simulink library "CAN_PT_lib"  (Simulink 7.5)
settings: Solver=ode45  StartTime=0.0  StopTime=10.0  RelTol=1e-3
undefined symbols (not defined in the file): p_bool_False_M, pOUTP_pct_BatSOCIC_CUR, pOUTP_pct_BatSOCLim_C, pOUTP_pct_BatSOCRaw_TAB, pOUTP_st_ACPTCfg_C, pOUTP_st_ChrgrPlugStOne_C, pOUTP_st_ChrgrPlugStTwo_C, pOUTP_st_ChrgrPlugStZero_C, pOUTP_st_DCDCErrSt_C, pOUTP_st_EVRdyNoSt_C, pOUTP_st_EVRdyRdySt_C, pOUTP_st_HCUStNoErr_C, pOUTP_w_OutPwrCvrt_C, pOUTP_w_OutPwrGenrMax_C, pOUTP_w_OutPwrMax_C, VMMCoorrStsTyp
libraries: BaseOperationLib_Browser x40, PES_CZ_FAW x1, simulink x1
settings Model: Creator=wuaibin  LastModifiedBy=wuaibin

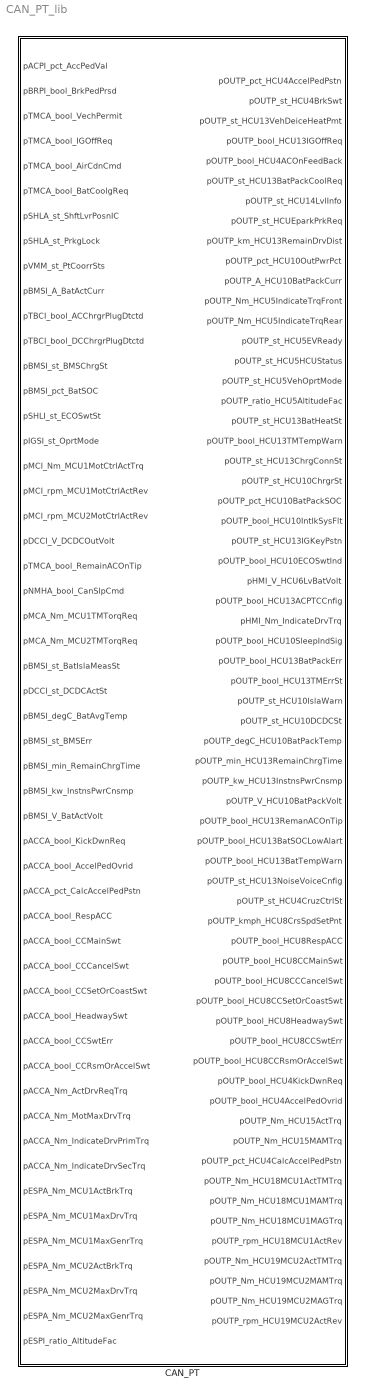
== system CAN_PT_lib ==
  CAN_PT : Subsystem  TreatAsAtomicUnit=on

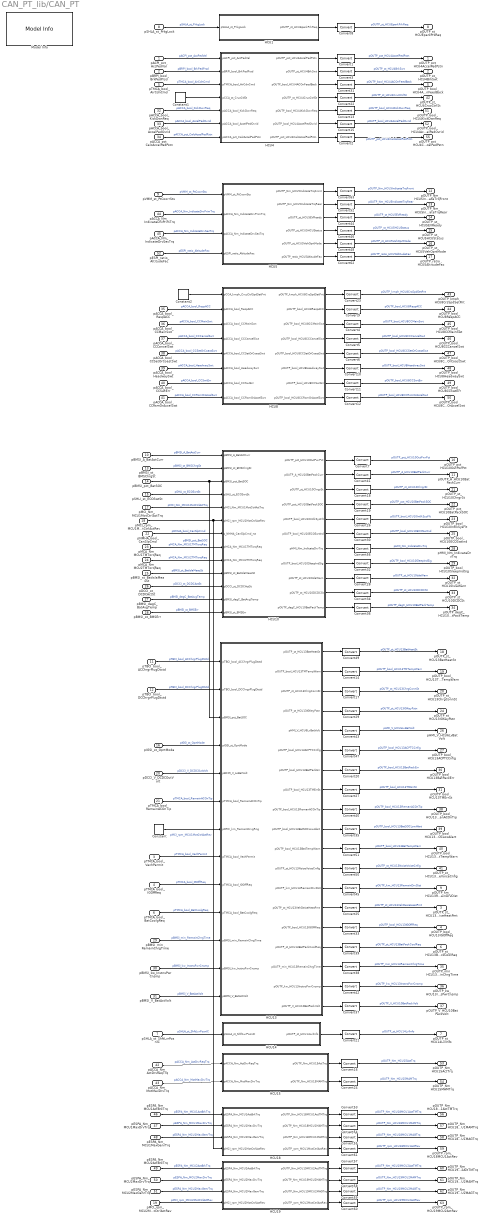
== system CAN_PT_lib/CAN_PT ==
  pACPI_pct_AccPedVal : Inport  OutDataType=fixdt(1, 16)  OutScaling=2^0
  pBRPI_bool_BrkPedPrsd : Inport  Port=2  OutDataType=fixdt(1, 16)  OutScaling=2^0
  pTMCA_bool_VechPermit : Inport  Port=3  OutDataType=fixdt(1, 16)  OutScaling=2^0
  pTMCA_bool_IGOffReq : Inport  Port=4  OutDataType=fixdt(1, 16)  OutScaling=2^0
  pTMCA_bool_AirCdnCmd : Inport  Port=5  OutDataType=fixdt(1, 16)  OutScaling=2^0
  pTMCA_bool_BatCoolgReq : Inport  Port=6  OutDataType=fixdt(1, 16)  OutScaling=2^0
  pSHLA_st_ShftLvrPosnIC : Inport  Port=7  OutDataType=fixdt(1, 16)  OutScaling=2^0
  pSHLA_st_PrkgLock : Inport  Port=8  OutDataType=fixdt(1, 16)  OutScaling=2^0
  pVMM_st_PtCoorrSts : Inport  Port=9
  pBMSI_A_BatActCurr : Inport  Port=10
  pTBCI_bool_ACChrgrPlugDtctd : Inport  Port=11
  pTBCI_bool_DCChrgrPlugDtctd : Inport  Port=12
  pBMSI_st_BMSChrgSt : Inport  Port=13
  pBMSI_pct_BatSOC : Inport  Port=14
  pSHLI_st_ECOSwtSt : Inport  Port=15
  pIGSI_st_OprtMode : Inport  Port=16
  pMCI_Nm_MCU1MotCtrlActTrq : Inport  Port=17
  pMCI_rpm_MCU1MotCtrlActRev : Inport  Port=18
  pMCI_rpm_MCU2MotCtrlActRev : Inport  Port=19
  pDCCI_V_DCDCOutVolt : Inport  Port=20
  pTMCA_bool_RemainACOnTip : Inport  Port=21
  pNMHA_bool_CanSlpCmd : Inport  Port=22  OutDataType=fixdt(1, 16)  OutScaling=2^0
  pMCA_Nm_MCU1TMTorqReq : Inport  Port=23
  pMCA_Nm_MCU2TMTorqReq : Inport  Port=24
  pBMSI_st_BatIslaMeasSt : Inport  Port=25
  pDCCI_st_DCDCActSt : Inport  Port=26
  pBMSI_degC_BatAvgTemp : Inport  Port=27
  pBMSI_st_BMSErr : Inport  Port=28
  pBMSI_min_RemainChrgTime : Inport  Port=29
  pBMSI_kw_InstnsPwrCnsmp : Inport  Port=30
  pBMSI_V_BatActVolt : Inport  Port=31
  pACCA_bool_KickDwnReq : Inport  Port=32  OutDataType=fixdt(1, 16)  OutScaling=2^0
  pACCA_bool_AccelPedOvrid : Inport  Port=33  OutDataType=fixdt(1, 16)  OutScaling=2^0
  pACCA_pct_CalcAccelPedPstn : Inport  Port=34  OutDataType=fixdt(1, 16)  OutScaling=2^0
  pACCA_bool_RespACC : Inport  Port=35
  pACCA_bool_CCMainSwt : Inport  Port=36
  pACCA_bool_CCCancelSwt : Inport  Port=37
  pACCA_bool_CCSetOrCoastSwt : Inport  Port=38
  pACCA_bool_HeadwaySwt : Inport  Port=39
  pACCA_bool_CCSwtErr : Inport  Port=40
  pACCA_bool_CCRsmOrAccelSwt : Inport  Port=41
  pACCA_Nm_ActDrvReqTrq : Inport  Port=42  OutDataType=fixdt(1, 16)  OutScaling=2^0
  pACCA_Nm_MotMaxDrvTrq : Inport  Port=43  OutDataType=fixdt(1, 16)  OutScaling=2^0
  pACCA_Nm_IndicateDrvPrimTrq : Inport  Port=44  OutDataType=fixdt(1, 16)  OutScaling=2^0
  pACCA_Nm_IndicateDrvSecTrq : Inport  Port=45  OutDataType=fixdt(1, 16)  OutScaling=2^0
  pESPA_Nm_MCU1ActBrkTrq : Inport  Port=46  OutDataType=fixdt(1, 16)  OutScaling=2^0
  pESPA_Nm_MCU1MaxDrvTrq : Inport  Port=47  OutDataType=fixdt(1, 16)  OutScaling=2^0
  pESPA_Nm_MCU1MaxGenrTrq : Inport  Port=48  OutDataType=fixdt(1, 16)  OutScaling=2^0
  pESPA_Nm_MCU2ActBrkTrq : Inport  Port=49  OutDataType=fixdt(1, 16)  OutScaling=2^0
  pESPA_Nm_MCU2MaxDrvTrq : Inport  Port=50  OutDataType=fixdt(1, 16)  OutScaling=2^0
  pESPA_Nm_MCU2MaxGenrTrq : Inport  Port=51  OutDataType=fixdt(1, 16)  OutScaling=2^0
  pESPI_ratio_AltitudeFac : Inport  Port=52  OutDataType=fixdt(1, 16)  OutScaling=2^0
  Constant : BaseOperationLib_Browser/Sources&Sinks/Constant  Value=0  OutMin=[]  OutMax=[]  OutDataType=fixdt(1, 16)  ConRadixGroup=Use specified scaling  OutScaling=2^0  OutDataTypeStr=Inherit: Inherit from 'Constant value'
  Constant1 : BaseOperationLib_Browser/Sources&Sinks/Constant  Value=0  OutMin=[]  OutMax=[]  OutDataType=fixdt(1, 16)  ConRadixGroup=Use specified scaling  OutScaling=2^0  OutDataTypeStr=Inherit: Inherit from 'Constant value'
  Constant2 : BaseOperationLib_Browser/Sources&Sinks/Constant  Value=0  OutMin=[]  OutMax=[]  OutDataType=fixdt(1, 16)  ConRadixGroup=Use specified scaling  OutScaling=2^0  OutDataTypeStr=Inherit: Inherit from 'Constant value'
  Convert{1..63} (63 alike) : DataTypeConversion  OutDataType=fixdt(1, 16)  OutScaling=2^0
  HCU1 : Subsystem
  HCU10 : Subsystem
  HCU13 : Subsystem
  HCU14 : Subsystem
  HCU15 : Subsystem
  HCU18 : Subsystem
  HCU19 : Subsystem
  HCU4 : Subsystem
  HCU5 : Subsystem
  HCU8 : Subsystem
  Model Info : simulink/Model-Wide Utilities/Model Info  SystemSampleTime=-1  InitialBlockCM=None  BlockCM=None  Frame=on  DisplayStringWithTags=Model Info\nCreated: %<Created>\nCreator: wuaibin  HorizontalTextAlignment=Center  LeftAlignmentValue=0.5  SourceBlockDiagram=HQEV_HCU  TagMaxNumber=20
  pOUTP_pct_HCU4AccelPedPstn : Outport  OutDataType=fixdt(1, 16)  OutScaling=2^0
  pOUTP_st_HCU4BrkSwt : Outport  Port=2  OutDataType=fixdt(1, 16)  OutScaling=2^0
  pOUTP_st_HCU13VehDeiceHeatPmt : Outport  Port=3  OutDataType=fixdt(1, 16)  OutScaling=2^0
  pOUTP_bool_HCU13IGOffReq : Outport  Port=4  OutDataType=fixdt(1, 16)  OutScaling=2^0
  pOUTP_bool_HCU4ACOnFeedBack : Outport  Port=5  OutDataType=fixdt(1, 16)  OutScaling=2^0
  pOUTP_st_HCU13BatPackCoolReq : Outport  Port=6  OutDataType=fixdt(1, 16)  OutScaling=2^0
  pOUTP_st_HCU14LvlInfo : Outport  Port=7  OutDataType=fixdt(1, 16)  OutScaling=2^0
  pOUTP_st_HCUEparkPrkReq : Outport  Port=8  OutDataType=fixdt(1, 16)  OutScaling=2^0
  pOUTP_km_HCU13RemainDrvDist : Outport  Port=9  OutDataType=fixdt(1, 16)  OutScaling=2^0
  pOUTP_pct_HCU10OutPwrPct : Outport  Port=10
  pOUTP_A_HCU10BatPackCurr : Outport  Port=11
  pOUTP_Nm_HCU5IndicateTrqFront : Outport  Port=12
  pOUTP_Nm_HCU5IndicateTrqRear : Outport  Port=13
  pOUTP_st_HCU5EVReady : Outport  Port=14
  pOUTP_st_HCU5HCUStatus : Outport  Port=15
  pOUTP_st_HCU5VehOprtMode : Outport  Port=16
  pOUTP_ratio_HCU5AltitudeFac : Outport  Port=17
  pOUTP_st_HCU13BatHeatSt : Outport  Port=18
  pOUTP_bool_HCU13TMTempWarn : Outport  Port=19
  pOUTP_st_HCU13ChrgConnSt : Outport  Port=20
  pOUTP_st_HCU10ChrgrSt : Outport  Port=21
  pOUTP_pct_HCU10BatPackSOC : Outport  Port=22
  pOUTP_bool_HCU10IntlkSysFlt : Outport  Port=23
  pOUTP_st_HCU13IGKeyPstn : Outport  Port=24
  pOUTP_bool_HCU10ECOSwtInd : Outport  Port=25
  pHMI_V_HCU6LvBatVolt : Outport  Port=26
  pOUTP_bool_HCU13ACPTCCnfig : Outport  Port=27
  pHMI_Nm_IndicateDrvTrq : Outport  Port=28
  pOUTP_bool_HCU10SleepIndSig : Outport  Port=29
  pOUTP_bool_HCU13BatPackErr : Outport  Port=30
  pOUTP_bool_HCU13TMErrSt : Outport  Port=31
  pOUTP_st_HCU10IslaWarn : Outport  Port=32
  pOUTP_st_HCU10DCDCSt : Outport  Port=33
  pOUTP_degC_HCU10BatPackTemp : Outport  Port=34
  pOUTP_min_HCU13RemainChrgTime : Outport  Port=35
  pOUTP_kw_HCU13InstnsPwrCnsmp : Outport  Port=36
  pOUTP_V_HCU10BatPackVolt : Outport  Port=37
  pOUTP_bool_HCU13RemanACOnTip : Outport  Port=38  OutDataType=fixdt(1, 16)  OutScaling=2^0
  pOUTP_bool_HCU13BatSOCLowAlart : Outport  Port=39
  pOUTP_bool_HCU13BatTempWarn : Outport  Port=40  OutDataType=fixdt(1, 16)  OutScaling=2^0
  pOUTP_st_HCU13NoiseVoiceCnfig : Outport  Port=41  OutDataType=fixdt(1, 16)  OutScaling=2^0
  pOUTP_st_HCU4CruzCtrlSt : Outport  Port=42  OutDataType=fixdt(1, 16)  OutScaling=2^0
  pOUTP_kmph_HCU8CrsSpdSetPnt : Outport  Port=43  OutDataType=fixdt(1, 16)  OutScaling=2^0
  pOUTP_bool_HCU8RespACC : Outport  Port=44  OutDataType=fixdt(1, 16)  OutScaling=2^0
  pOUTP_bool_HCU8CCMainSwt : Outport  Port=45  OutDataType=fixdt(1, 16)  OutScaling=2^0
  pOUTP_bool_HCU8CCCancelSwt : Outport  Port=46  OutDataType=fixdt(1, 16)  OutScaling=2^0
  pOUTP_bool_HCU8CCSetOrCoastSwt : Outport  Port=47  OutDataType=fixdt(1, 16)  OutScaling=2^0
  pOUTP_bool_HCU8HeadwaySwt : Outport  Port=48  OutDataType=fixdt(1, 16)  OutScaling=2^0
  pOUTP_bool_HCU8CCSwtErr : Outport  Port=49  OutDataType=fixdt(1, 16)  OutScaling=2^0
  pOUTP_bool_HCU8CCRsmOrAccelSwt : Outport  Port=50  OutDataType=fixdt(1, 16)  OutScaling=2^0
  pOUTP_bool_HCU4KickDwnReq : Outport  Port=51
  pOUTP_bool_HCU4AccelPedOvrid : Outport  Port=52
  pOUTP_Nm_HCU15ActTrq : Outport  Port=53
  pOUTP_Nm_HCU15MAMTrq : Outport  Port=54
  pOUTP_pct_HCU4CalcAccelPedPstn : Outport  Port=55  OutDataType=fixdt(1, 16)  OutScaling=2^0
  pOUTP_Nm_HCU18MCU1ActTMTrq : Outport  Port=56
  pOUTP_Nm_HCU18MCU1MAMTrq : Outport  Port=57
  pOUTP_Nm_HCU18MCU1MAGTrq : Outport  Port=58
  pOUTP_rpm_HCU18MCU1ActRev : Outport  Port=59
  pOUTP_Nm_HCU19MCU2ActTMTrq : Outport  Port=60
  pOUTP_Nm_HCU19MCU2MAMTrq : Outport  Port=61
  pOUTP_Nm_HCU19MCU2MAGTrq : Outport  Port=62
  pOUTP_rpm_HCU19MCU2ActRev : Outport  Port=63
  wires:
  HCU15/2(pOUTP_Nm_HCU15MAMTrq) -> Convert24/1
  HCU15/1(pOUTP_Nm_HCU15ActTrq) -> Convert16/1
  HCU4/7(pOUTP_pct_HCU4CalcAccelPedPstn) -> Convert2/1
  HCU4/6(pOUTP_bool_HCU4AccelPedOvrid) -> Convert15/1
  HCU4/5(pOUTP_bool_HCU4KickDwnReq) -> Convert13/1
  HCU4/4(pOUTP_st_HCU4CruzCtrlSt) -> Convert22/1
  HCU13/19(pOUTP_V_HCU10BatPackVolt) -> Convert37/1
  HCU13/18(pOUTP_kw_HCU13InstnsPwrCnsmp) -> Convert42/1
  HCU13/17(pOUTP_min_HCU13RemainChrgTime) -> Convert38/1
  HCU10/11(pOUTP_degC_HCU10BatPackTemp) -> Convert36/1
  HCU10/10(pOUTP_st_HCU10DCDCSt) -> Convert34/1
  HCU10/9(pOUTP_st_HCU10IslaWarn) -> Convert28/1
  Constant/1 -> HCU13/7(pDRC_km_RemainDrvgRng)
  Convert49/1 -> pOUTP_st_HCU13BatHeatSt/1  "pOUTP_st_HCU13BatHeatSt"
  Convert14/1 -> pOUTP_bool_HCU13TMTempWarn/1  "pOUTP_bool_HCU13TMTempWarn"
  Convert17/1 -> pOUTP_st_HCU13ChrgConnSt/1  "pOUTP_st_HCU13ChrgConnSt"
  HCU13/5(pHMI_V_HCU6LvBatVolt) -> Convert43/1
  HCU5/5(pOUTP_st_HCU5VehOprtMode) -> Convert48/1
  HCU5/4(pOUTP_st_HCU5HCUStatus) -> Convert46/1
  HCU5/3(pOUTP_st_HCU5EVReady) -> Convert44/1
  HCU13/6(pOUTP_bool_HCU13ACPTCCnfig) -> Convert47/1
  HCU13/4(pOUTP_st_HCU13IGKeyPstn) -> Convert29/1
  HCU13/3(pOUTP_st_HCU13ChrgConnSt) -> Convert17/1
  HCU13/2(pOUTP_bool_HCU13TMTempWarn) -> Convert14/1
  HCU13/1(pOUTP_st_HCU13BatHeatSt) -> Convert49/1
  HCU13/13(pOUTP_km_HCU13RemainDrvDist) -> Convert45/1
  HCU13/12(pOUTP_st_HCU13NoiseVoiceCnfig) -> Convert50/1
  HCU13/11(pOUTP_bool_HCU13BatTempWarn) -> Convert51/1
  HCU13/10(pOUTP_bool_HCU13BatSOCLowAlart) -> Convert35/1
  HCU13/9(pOUTP_bool_HCU13RemanACOnTip) -> Convert40/1
  HCU13/8(pOUTP_bool_HCU13TMErrSt) -> Convert27/1
  HCU13/7(pOUTP_bool_HCU13BatPackErr) -> Convert20/1
  pSHLA_st_PrkgLock/1 -> HCU1/1(pSHLA_st_PrkgLock)  "pSHLA_st_PrkgLock"
  HCU1/1(pOUTP_st_HCUEparkPrkReq) -> Convert8/1
  pSHLA_st_ShftLvrPosnIC/1 -> HCU14/1(pSHLA_st_ShftLvrPosnIC)  "pSHLA_st_ShftLvrPosnIC"
  HCU14/1(pOUTP_st_HCU14LvlInfo) -> Convert21/1
  pTMCA_bool_AirCdnCmd/1 -> HCU4/3(pTMCA_bool_AirCdnCmd)  "pTMCA_bool_AirCdnCmd"
  HCU4/3(pOUTP_bool_HCU4ACOnFeedBack) -> Convert31/1
  pBRPI_bool_BrkPedPrsd/1 -> HCU4/2(pBRPI_bool_BrkPedPrsd)  "pBRPI_bool_BrkPedPrsd"
  pACPI_pct_AccPedVal/1 -> HCU4/1(pACPI_pct_AccPedVal)  "pACPI_pct_AccPedVal"
  HCU4/2(pOUTP_st_HCU4BrkSwt) -> Convert3/1
  HCU4/1(pOUTP_pct_HCU4AccelPedPstn) -> Convert1/1
  pMCA_Nm_MCU1TMTorqReq/1 -> HCU10/8(pMCA_Nm_MCU1TMTorqReq)  "pMCA_Nm_MCU1TMTorqReq"
  pMCA_Nm_MCU2TMTorqReq/1 -> HCU10/9(pMCA_Nm_MCU2TMTorqReq)  "pMCA_Nm_MCU2TMTorqReq"
  Constant2/1 -> HCU8/1(pCCA_kmph_CruzCtrlSpdSetPnt)
  Convert2/1 -> pOUTP_pct_HCU4CalcAccelPedPstn/1  "pOUTP_pct_HCU4CalcAccelPedPstn"
  Convert24/1 -> pOUTP_Nm_HCU15MAMTrq/1  "pOUTP_Nm_HCU15MAMTrq"
  Convert16/1 -> pOUTP_Nm_HCU15ActTrq/1  "pOUTP_Nm_HCU15ActTrq"
  Convert15/1 -> pOUTP_bool_HCU4AccelPedOvrid/1  "pOUTP_bool_HCU4AccelPedOvrid"
  Convert13/1 -> pOUTP_bool_HCU4KickDwnReq/1  "pOUTP_bool_HCU4KickDwnReq"
  HCU8/8(pOUTP_bool_HCU8CCRsmOrAccelSwt) -> Convert12/1
  HCU8/7(pOUTP_bool_HCU8CCSwtErr) -> Convert11/1
  HCU8/6(pOUTP_bool_HCU8HeadwaySwt) -> Convert10/1
  HCU8/5(pOUTP_bool_HCU8CCSetOrCoastSwt) -> Convert6/1
  HCU8/4(pOUTP_bool_HCU8CCCancelSwt) -> Convert5/1
  HCU8/3(pOUTP_bool_HCU8CCMainSwt) -> Convert4/1
  HCU8/2(pOUTP_bool_HCU8RespACC) -> Convert9/1
  HCU8/1(pOUTP_kmph_HCU8CrsSpdSetPnt) -> Convert23/1
  Convert6/1 -> pOUTP_bool_HCU8CCSetOrCoastSwt/1  "pOUTP_bool_HCU8CCSetOrCoastSwt"
  Convert5/1 -> pOUTP_bool_HCU8CCCancelSwt/1  "pOUTP_bool_HCU8CCCancelSwt"
  Convert4/1 -> pOUTP_bool_HCU8CCMainSwt/1  "pOUTP_bool_HCU8CCMainSwt"
  Convert12/1 -> pOUTP_bool_HCU8CCRsmOrAccelSwt/1  "pOUTP_bool_HCU8CCRsmOrAccelSwt"
  Convert11/1 -> pOUTP_bool_HCU8CCSwtErr/1  "pOUTP_bool_HCU8CCSwtErr"
  Convert10/1 -> pOUTP_bool_HCU8HeadwaySwt/1  "pOUTP_bool_HCU8HeadwaySwt"
  Convert9/1 -> pOUTP_bool_HCU8RespACC/1  "pOUTP_bool_HCU8RespACC"
  Convert23/1 -> pOUTP_kmph_HCU8CrsSpdSetPnt/1  "pOUTP_kmph_HCU8CrsSpdSetPnt"
  Convert22/1 -> pOUTP_st_HCU4CruzCtrlSt/1  "pOUTP_st_HCU4CruzCtrlSt"
  Convert51/1 -> pOUTP_bool_HCU13BatTempWarn/1  "pOUTP_bool_HCU13BatTempWarn"
  Convert50/1 -> pOUTP_st_HCU13NoiseVoiceCnfig/1  "pOUTP_st_HCU13NoiseVoiceCnfig"
  Convert35/1 -> pOUTP_bool_HCU13BatSOCLowAlart/1  "pOUTP_bool_HCU13BatSOCLowAlart"
  HCU10/7(pHMI_Nm_IndicateDrvTrq) -> Convert56/1
  Convert56/1 -> pHMI_Nm_IndicateDrvTrq/1  "pHMI_Nm_IndicateDrvTrq"
  HCU10/1(pOUTP_pct_HCU10OutPwrPct) -> Convert7/1
  Convert7/1 -> pOUTP_pct_HCU10OutPwrPct/1  "pOUTP_pct_HCU10OutPwrPct"
  Convert41/1 -> pOUTP_A_HCU10BatPackCurr/1  "pOUTP_A_HCU10BatPackCurr"
  HCU10/2(pOUTP_A_HCU10BatPackCurr) -> Convert41/1
  Convert44/1 -> pOUTP_st_HCU5EVReady/1  "pOUTP_st_HCU5EVReady"
  Convert46/1 -> pOUTP_st_HCU5HCUStatus/1  "pOUTP_st_HCU5HCUStatus"
  Convert48/1 -> pOUTP_st_HCU5VehOprtMode/1  "pOUTP_st_HCU5VehOprtMode"
  HCU10/3(pOUTP_st_HCU10ChrgrSt) -> Convert18/1
  Convert18/1 -> pOUTP_st_HCU10ChrgrSt/1  "pOUTP_st_HCU10ChrgrSt"
  HCU10/4(pOUTP_pct_HCU10BatPackSOC) -> Convert19/1
  Convert19/1 -> pOUTP_pct_HCU10BatPackSOC/1  "pOUTP_pct_HCU10BatPackSOC"
  Convert26/1 -> pOUTP_bool_HCU10IntlkSysFlt/1  "pOUTP_bool_HCU10IntlkSysFlt"
  HCU10/5(pOUTP_bool_HCU10IntlkSysFlt) -> Convert26/1
  Convert29/1 -> pOUTP_st_HCU13IGKeyPstn/1  "pOUTP_st_HCU13IGKeyPstn"
  Convert30/1 -> pOUTP_bool_HCU10ECOSwtInd/1  "pOUTP_bool_HCU10ECOSwtInd"
  HCU10/6(pOUTP_bool_HCU10ECOSwtInd) -> Convert30/1
  Convert43/1 -> pHMI_V_HCU6LvBatVolt/1  "pHMI_V_HCU6LvBatVolt"
  Convert47/1 -> pOUTP_bool_HCU13ACPTCCnfig/1  "pOUTP_bool_HCU13ACPTCCnfig"
  pVMM_st_PtCoorrSts/1 -> HCU5/1(pVMM_st_PtCoorrSts)  "pVMM_st_PtCoorrSts"
  pBMSI_A_BatActCurr/1 -> HCU10/1(pBMSI_A_BatActCurr)  "pBMSI_A_BatActCurr"
  pTBCI_bool_ACChrgrPlugDtctd/1 -> HCU13/1(pTBCI_bool_ACChrgrPlugDtctd)  "pTBCI_bool_ACChrgrPlugDtctd"
  pTBCI_bool_DCChrgrPlugDtctd/1 -> HCU13/2(pTBCI_bool_DCChrgrPlugDtctd)  "pTBCI_bool_DCChrgrPlugDtctd"
  pBMSI_st_BMSChrgSt/1 -> HCU10/2(pBMSI_st_BMSChrgSt)  "pBMSI_st_BMSChrgSt"
  pBMSI_pct_BatSOC/1 -> HCU13/3(pBMSI_pct_BatSOC), HCU10/3(pBMSI_pct_BatSOC)  "pBMSI_pct_BatSOC"
  pSHLI_st_ECOSwtSt/1 -> HCU10/4(pSHLI_st_ECOSwtSt)  "pSHLI_st_ECOSwtSt"
  pIGSI_st_OprtMode/1 -> HCU13/4(pIGSI_st_OprtMode)  "pIGSI_st_OprtMode"
  pDCCI_V_DCDCOutVolt/1 -> HCU13/5(pBCMI_V_LoBatVolt)  "pDCCI_V_DCDCOutVolt"
  pMCI_Nm_MCU1MotCtrlActTrq/1 -> HCU10/5(pMCI_Nm_MCU1MotCtrlActTrq)  "pMCI_Nm_MCU1MotCtrlActTrq"
  pMCI_rpm_MCU1MotCtrlActRev/1 -> HCU10/6(pMCI_rpm_MCU1MotCtrlActRev), HCU18/4(pMCI_rpm_MCU1MotCtrlActRev)  "pMCI_rpm_MCU1MotCtrlActRev"
  Convert32/1 -> pOUTP_bool_HCU10SleepIndSig/1  "pOUTP_bool_HCU10SleepIndSig"
  HCU10/8(pOUTP_bool_HCU10SleepIndSig) -> Convert32/1
  pNMHA_bool_CanSlpCmd/1 -> HCU10/7(s_NMHA_CanSlpCmd_na)  "pNMHA_bool_CanSlpCmd"
  Convert20/1 -> pOUTP_bool_HCU13BatPackErr/1  "pOUTP_bool_HCU13BatPackErr"
  Convert27/1 -> pOUTP_bool_HCU13TMErrSt/1  "pOUTP_bool_HCU13TMErrSt"
  pBMSI_st_BatIslaMeasSt/1 -> HCU10/10(pBMSI_st_BatIslaMeasSt)  "pBMSI_st_BatIslaMeasSt"
  pDCCI_st_DCDCActSt/1 -> HCU10/11(pDCCI_st_DCDCActSt)  "pDCCI_st_DCDCActSt"
  pBMSI_degC_BatAvgTemp/1 -> HCU10/12(pBMSI_degC_BatAvgTemp)  "pBMSI_degC_BatAvgTemp"
  Convert34/1 -> pOUTP_st_HCU10DCDCSt/1  "pOUTP_st_HCU10DCDCSt"
  Convert36/1 -> pOUTP_degC_HCU10BatPackTemp/1  "pOUTP_degC_HCU10BatPackTemp"
  Convert28/1 -> pOUTP_st_HCU10IslaWarn/1  "pOUTP_st_HCU10IslaWarn"
  pBMSI_min_RemainChrgTime/1 -> HCU13/11(pBMSI_min_RemainChrgTime)  "pBMSI_min_RemainChrgTime"
  pBMSI_kw_InstnsPwrCnsmp/1 -> HCU13/12(pBMSI_kw_InstnsPwrCnsmp)  "pBMSI_kw_InstnsPwrCnsmp"
  Convert38/1 -> pOUTP_min_HCU13RemainChrgTime/1  "pOUTP_min_HCU13RemainChrgTime"
  Convert42/1 -> pOUTP_kw_HCU13InstnsPwrCnsmp/1  "pOUTP_kw_HCU13InstnsPwrCnsmp"
  pBMSI_V_BatActVolt/1 -> HCU13/13(pBMSI_V_BatActVolt)  "pBMSI_V_BatActVolt"
  Convert37/1 -> pOUTP_V_HCU10BatPackVolt/1  "pOUTP_V_HCU10BatPackVolt"
  Convert40/1 -> pOUTP_bool_HCU13RemanACOnTip/1  "pOUTP_bool_HCU13RemanACOnTip"
  pTMCA_bool_RemainACOnTip/1 -> HCU13/6(pTMCA_bool_RemainACOnTip)  "pTMCA_bool_RemainACOnTip"
  Convert45/1 -> pOUTP_km_HCU13RemainDrvDist/1  "pOUTP_km_HCU13RemainDrvDist"
  HCU13/16(pOUTP_st_HCU13BatPackCoolReq) -> Convert39/1
  Convert39/1 -> pOUTP_st_HCU13BatPackCoolReq/1  "pOUTP_st_HCU13BatPackCoolReq"
  pTMCA_bool_BatCoolgReq/1 -> HCU13/10(pTMCA_bool_BatCoolgReq)  "pTMCA_bool_BatCoolgReq"
  Convert31/1 -> pOUTP_bool_HCU4ACOnFeedBack/1  "pOUTP_bool_HCU4ACOnFeedBack"
  Convert21/1 -> pOUTP_st_HCU14LvlInfo/1  "pOUTP_st_HCU14LvlInfo"
  Convert8/1 -> pOUTP_st_HCUEparkPrkReq/1  "pOUTP_st_HCUEparkPrkReq"
  Convert3/1 -> pOUTP_st_HCU4BrkSwt/1  "pOUTP_st_HCU4BrkSwt"
  Convert1/1 -> pOUTP_pct_HCU4AccelPedPstn/1  "pOUTP_pct_HCU4AccelPedPstn"
  HCU13/14(pOUTP_st_HCU13VehDeiceHeatPmt) -> Convert25/1
  HCU13/15(pOUTP_bool_HCU13IGOffReq) -> Convert33/1
  pTMCA_bool_VechPermit/1 -> HCU13/8(pTMCA_bool_VechPermit)  "pTMCA_bool_VechPermit"
  pTMCA_bool_IGOffReq/1 -> HCU13/9(pTMCA_bool_IGOffReq)  "pTMCA_bool_IGOffReq"
  Convert25/1 -> pOUTP_st_HCU13VehDeiceHeatPmt/1  "pOUTP_st_HCU13VehDeiceHeatPmt"
  Convert33/1 -> pOUTP_bool_HCU13IGOffReq/1  "pOUTP_bool_HCU13IGOffReq"
  pACCA_bool_KickDwnReq/1 -> HCU4/5(pACCA_bool_KickDwnReq)  "pACCA_bool_KickDwnReq"
  pACCA_bool_AccelPedOvrid/1 -> HCU4/6(pACCA_bool_AccelPedOvrid)  "pACCA_bool_AccelPedOvrid"
  pACCA_pct_CalcAccelPedPstn/1 -> HCU4/7(pACCA_pct_CalcAccelPedPstn)  "pACCA_pct_CalcAccelPedPstn"
  Constant1/1 -> HCU4/4(pCCA_st_CruzCtlSt)
  pACCA_bool_RespACC/1 -> HCU8/2(pACCA_bool_RespACC)  "pACCA_bool_RespACC"
  pACCA_bool_CCMainSwt/1 -> HCU8/3(pACCA_bool_CCMainSwt)  "pACCA_bool_CCMainSwt"
  pACCA_bool_CCCancelSwt/1 -> HCU8/4(pACCA_bool_CCCancelSwt)  "pACCA_bool_CCCancelSwt"
  pACCA_bool_CCSetOrCoastSwt/1 -> HCU8/5(pACCA_bool_CCSetOrCoastSwt)  "pACCA_bool_CCSetOrCoastSwt"
  pACCA_bool_HeadwaySwt/1 -> HCU8/6(pACCA_bool_HeadwaySwt)  "pACCA_bool_HeadwaySwt"
  pACCA_bool_CCSwtErr/1 -> HCU8/7(pACCA_bool_CCSwtErr)  "pACCA_bool_CCSwtErr"
  pACCA_bool_CCRsmOrAccelSwt/1 -> HCU8/8(pACCA_bool_CCRsmOrAccelSwt)  "pACCA_bool_CCRsmOrAccelSwt"
  pACCA_Nm_ActDrvReqTrq/1 -> HCU15/1(pACCA_Nm_ActDrvReqTrq)  "pACCA_Nm_ActDrvReqTrq"
  pACCA_Nm_MotMaxDrvTrq/1 -> HCU15/2(pACCA_Nm_MotMaxDrvTrq)  "pACCA_Nm_MotMaxDrvTrq"
  pACCA_Nm_IndicateDrvPrimTrq/1 -> HCU5/2(pACCA_Nm_IndicateDrvPrimTrq)  "pACCA_Nm_IndicateDrvPrimTrq"
  HCU18/1(pOUTP_Nm_HCU18MCU1ActTMTrq) -> Convert53/1
  HCU18/2(pOUTP_Nm_HCU18MCU1MAMTrq) -> Convert54/1
  HCU18/3(pOUTP_Nm_HCU18MCU1MAGTrq) -> Convert55/1
  Convert53/1 -> pOUTP_Nm_HCU18MCU1ActTMTrq/1  "pOUTP_Nm_HCU18MCU1ActTMTrq"
  Convert54/1 -> pOUTP_Nm_HCU18MCU1MAMTrq/1  "pOUTP_Nm_HCU18MCU1MAMTrq"
  Convert55/1 -> pOUTP_Nm_HCU18MCU1MAGTrq/1  "pOUTP_Nm_HCU18MCU1MAGTrq"
  HCU19/1(pOUTP_Nm_HCU19MCU2ActTMTrq) -> Convert57/1
  HCU19/2(pOUTP_Nm_HCU19MCU2MAMTrq) -> Convert58/1
  HCU19/3(pOUTP_Nm_HCU19MCU2MAGTrq) -> Convert59/1
  Convert57/1 -> pOUTP_Nm_HCU19MCU2ActTMTrq/1  "pOUTP_Nm_HCU19MCU2ActTMTrq"
  Convert58/1 -> pOUTP_Nm_HCU19MCU2MAMTrq/1  "pOUTP_Nm_HCU19MCU2MAMTrq"
  Convert59/1 -> pOUTP_Nm_HCU19MCU2MAGTrq/1  "pOUTP_Nm_HCU19MCU2MAGTrq"
  pESPA_Nm_MCU1ActBrkTrq/1 -> HCU18/1(pESPA_Nm_MCU1ActBrkTrq)  "pESPA_Nm_MCU1ActBrkTrq"
  pESPA_Nm_MCU1MaxDrvTrq/1 -> HCU18/2(pESPA_Nm_MCU1MaxDrvTrq)  "pESPA_Nm_MCU1MaxDrvTrq"
  pESPA_Nm_MCU1MaxGenrTrq/1 -> HCU18/3(pESPA_Nm_MCU1MaxGenrTrq)  "pESPA_Nm_MCU1MaxGenrTrq"
  pESPA_Nm_MCU2ActBrkTrq/1 -> HCU19/1(pESPA_Nm_MCU2ActBrkTrq)  "pESPA_Nm_MCU2ActBrkTrq"
  pESPA_Nm_MCU2MaxDrvTrq/1 -> HCU19/2(pESPA_Nm_MCU2MaxDrvTrq)  "pESPA_Nm_MCU2MaxDrvTrq"
  pESPA_Nm_MCU2MaxGenrTrq/1 -> HCU19/3(pESPA_Nm_MCU2MaxGenrTrq)  "pESPA_Nm_MCU2MaxGenrTrq"
  pBMSI_st_BMSErr/1 -> HCU10/13(pBMSI_st_BMSErr)  "pBMSI_st_BMSErr"
  pMCI_rpm_MCU2MotCtrlActRev/1 -> HCU19/4(pMCI_rpm_MCU2MotCtrlActRev)  "pMCI_rpm_MCU2MotCtrlActRev"
  Convert60/1 -> pOUTP_rpm_HCU19MCU2ActRev/1  "pOUTP_rpm_HCU19MCU2ActRev"
  Convert61/1 -> pOUTP_rpm_HCU18MCU1ActRev/1  "pOUTP_rpm_HCU18MCU1ActRev"
  HCU18/4(pOUTP_rpm_MCU1MotCtrlActRev) -> Convert61/1
  HCU19/4(pOUTP_rpm_MCU2MotCtrlActRev) -> Convert60/1
  Convert62/1 -> pOUTP_ratio_HCU5AltitudeFac/1  "pOUTP_ratio_HCU5AltitudeFac"
  HCU5/6(pOUTP_ratio_HCU5AltitudeFac) -> Convert62/1
  HCU5/2(pOUTP_Nm_HCU5IndicateTrqRear) -> Convert52/1
  Convert52/1 -> pOUTP_Nm_HCU5IndicateTrqRear/1  "pOUTP_Nm_HCU5IndicateTrqRear"
  HCU5/1(pOUTP_Nm_HCU5IndicateTrqFront) -> Convert63/1
  Convert63/1 -> pOUTP_Nm_HCU5IndicateTrqFront/1  "pOUTP_Nm_HCU5IndicateTrqFront"
  pACCA_Nm_IndicateDrvSecTrq/1 -> HCU5/3(pACCA_Nm_IndicateDrvSecTrq)  "pACCA_Nm_IndicateDrvSecTrq"
  pESPI_ratio_AltitudeFac/1 -> HCU5/4(pESPI_ratio_AltitudeFac)  "pESPI_ratio_AltitudeFac"

== system CAN_PT_lib/CAN_PT/HCU1 ==
  pSHLA_st_PrkgLock : Inport  OutDataType=fixdt(1, 16)  OutScaling=2^0
  pOUTP_st_HCUEparkPrkReq : Outport  OutDataType=fixdt(1, 16)  OutScaling=2^0
  wires:
  pSHLA_st_PrkgLock/1 -> pOUTP_st_HCUEparkPrkReq/1  "pSHLA_st_PrkgLock"

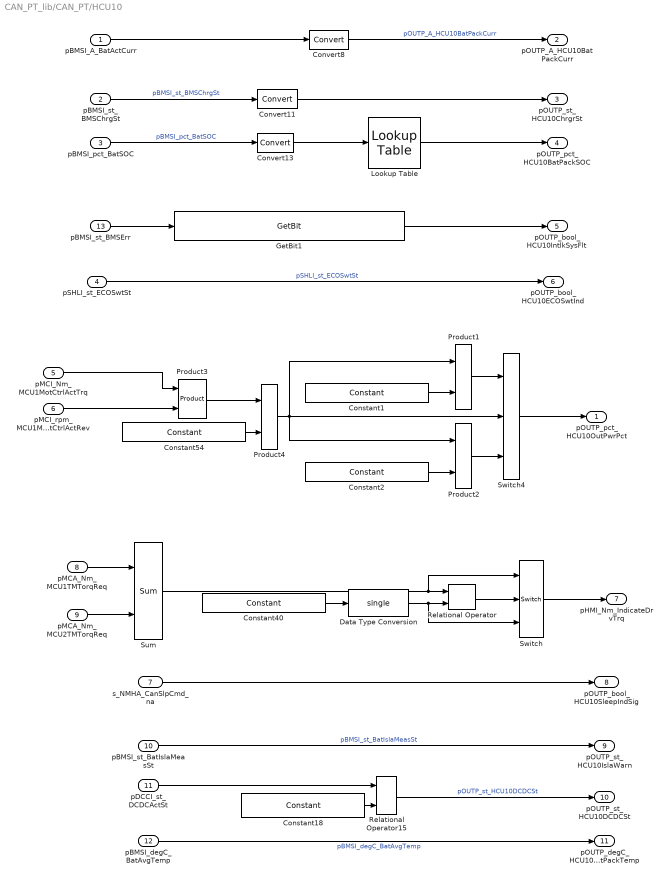
== system CAN_PT_lib/CAN_PT/HCU10 ==
  pBMSI_A_BatActCurr : Inport
  pBMSI_st_BMSChrgSt : Inport  Port=2
  pBMSI_pct_BatSOC : Inport  Port=3
  pSHLI_st_ECOSwtSt : Inport  Port=4
  pMCI_Nm_MCU1MotCtrlActTrq : Inport  Port=5
  pMCI_rpm_MCU1MotCtrlActRev : Inport  Port=6
  s_NMHA_CanSlpCmd_na : Inport  Port=7  OutDataType=fixdt(1, 16)  OutScaling=2^0
  pMCA_Nm_MCU1TMTorqReq : Inport  Port=8
  pMCA_Nm_MCU2TMTorqReq : Inport  Port=9
  pBMSI_st_BatIslaMeasSt : Inport  Port=10
  pDCCI_st_DCDCActSt : Inport  Port=11
  pBMSI_degC_BatAvgTemp : Inport  Port=12
  pBMSI_st_BMSErr : Inport  Port=13
  Constant1 : BaseOperationLib_Browser/Sources&Sinks/Constant  Value=pOUTP_w_OutPwrMax_C  OutMin=[]  OutMax=[]  OutDataType=fixdt(1, 16)  ConRadixGroup=Use specified scaling  OutScaling=2^0  OutDataTypeStr=Inherit: Inherit from 'Constant value'
  Constant18 : BaseOperationLib_Browser/Sources&Sinks/Constant  Value=pOUTP_st_DCDCErrSt_C  OutMin=[]  OutMax=[]  OutDataType=fixdt(1, 16)  ConRadixGroup=Use specified scaling  OutScaling=2^0  OutDataTypeStr=Inherit: Inherit from 'Constant value'
  Constant2 : BaseOperationLib_Browser/Sources&Sinks/Constant  Value=pOUTP_w_OutPwrGenrMax_C  OutMin=[]  OutMax=[]  OutDataType=fixdt(1, 16)  ConRadixGroup=Use specified scaling  OutScaling=2^0  OutDataTypeStr=Inherit: Inherit from 'Constant value'
  Constant40 : BaseOperationLib_Browser/Sources&Sinks/Constant  Value=p_bool_False_M  OutMin=[]  OutMax=[]  OutDataType=fixdt(1, 16)  ConRadixGroup=Use specified scaling  OutScaling=2^0  OutDataTypeStr=Inherit: Inherit from 'Constant value'
  Constant54 : BaseOperationLib_Browser/Sources&Sinks/Constant  Value=pOUTP_w_OutPwrCvrt_C  OutMin=[]  OutMax=[]  OutDataType=fixdt(1, 16)  ConRadixGroup=Use specified scaling  OutScaling=2^0  OutDataTypeStr=Inherit: Inherit from 'Constant value'
  Convert11 : DataTypeConversion  OutDataType=fixdt(1, 16)  OutScaling=2^0
  Convert13 : DataTypeConversion  OutDataType=fixdt(1, 16)  OutScaling=2^0
  Convert8 : DataTypeConversion  OutDataType=fixdt(1, 16)  OutScaling=2^0
  Data Type Conversion : DataTypeConversion  OutDataTypeMode=single  OutDataType=fixdt(1, 16)  OutScaling=2^0  OutDataTypeStr=single
  GetBit1 : PES_CZ_FAW/Discontinuities/GetBit  SystemSampleTime=-1  maska=FAWBmsErrTyp.InterLockErr
  Lookup Table : BaseOperationLib_Browser/Lookup Tables Changed/Lookup Table  InputValues=pOUTP_pct_BatSOCRaw_TAB  Table=pOUTP_pct_BatSOCIC_CUR  LookUpMeth=Interpolation-Use End Values  OutMin=[]  OutMax=[]  OutDataType=fixdt(1, 16)  OutScaling=2^0  OutDataTypeStr=Inherit: Inherit via back propagation  SaturateOnIntegerOverflow=on
      settings: AttributesFormatString=X:%<InputValues>\nTAB:%<Table>
  Product1 : BaseOperationLib_Browser/Math Operations Changed/Product  Inputs=*/  Multiplication=Element-wise(.*)  OutMin=[]  OutMax=[]  OutDataType=fixdt(1,16,0)  OutScaling=[]  OutDataTypeStr=Inherit: Inherit via back propagation  RndMeth=Zero  SaturateOnIntegerOverflow=on
  Product2 : BaseOperationLib_Browser/Math Operations Changed/Product  Inputs=*/  Multiplication=Element-wise(.*)  OutMin=[]  OutMax=[]  OutDataType=fixdt(1,16,0)  OutScaling=[]  OutDataTypeStr=Inherit: Inherit via back propagation  RndMeth=Zero  SaturateOnIntegerOverflow=on
  Product3 : BaseOperationLib_Browser/Math Operations Changed/Product  Inputs=2  Multiplication=Element-wise(.*)  OutMin=[]  OutMax=[]  OutDataType=fixdt(1,16,0)  OutScaling=[]  OutDataTypeStr=Inherit: Inherit via back propagation  RndMeth=Zero  SaturateOnIntegerOverflow=on
  Product4 : BaseOperationLib_Browser/Math Operations Changed/Product  Inputs=*/  Multiplication=Element-wise(.*)  OutMin=[]  OutMax=[]  OutDataType=fixdt(1,16,0)  OutScaling=[]  OutDataTypeStr=Inherit: Inherit via back propagation  RndMeth=Zero  SaturateOnIntegerOverflow=on
  Relational Operator : BaseOperationLib_Browser/Logic Operations Changed/Relational Operator  Operator=>=  InputSameDT=on  LogicOutDataTypeMode=Specify via dialog  LogicDataType=PDT_Bool  OutDataTypeStr=PDT_Bool
  Relational Operator15 : BaseOperationLib_Browser/Logic Operations Changed/Relational Operator  Operator===  InputSameDT=on  LogicOutDataTypeMode=Specify via dialog  LogicDataType=PDT_Bool  OutDataTypeStr=PDT_Bool
  Sum : BaseOperationLib_Browser/Math Operations Changed/Sum  Inputs=++  InputSameDT=on  OutMin=[]  OutMax=[]  OutDataType=fixdt(1, 16)  OutScaling=2^0  SaturateOnIntegerOverflow=on
  Switch : BaseOperationLib_Browser/Signal Routing Changed/Switch  Criteria=u2 ~= 0  Threshold=1  InputSameDT=on  OutMin=[]  OutMax=[]  OutDataType=fixdt(1,16,0)  OutScaling=[]  SaturateOnIntegerOverflow=on
  Switch4 : BaseOperationLib_Browser/Signal Routing Changed/Switch  Criteria=u2 >= Threshold  Threshold=0  InputSameDT=on  OutMin=[]  OutMax=[]  OutDataType=fixdt(1,16,0)  OutScaling=[]  SaturateOnIntegerOverflow=on
  pOUTP_pct_HCU10OutPwrPct : Outport
  pOUTP_A_HCU10BatPackCurr : Outport  Port=2
  pOUTP_st_HCU10ChrgrSt : Outport  Port=3
  pOUTP_pct_HCU10BatPackSOC : Outport  Port=4
  pOUTP_bool_HCU10IntlkSysFlt : Outport  Port=5
  pOUTP_bool_HCU10ECOSwtInd : Outport  Port=6
  pHMI_Nm_IndicateDrvTrq : Outport  Port=7
  pOUTP_bool_HCU10SleepIndSig : Outport  Port=8  OutDataType=fixdt(1, 16)  OutScaling=2^0
  pOUTP_st_HCU10IslaWarn : Outport  Port=9
  pOUTP_st_HCU10DCDCSt : Outport  Port=10
  pOUTP_degC_HCU10BatPackTemp : Outport  Port=11
  wires:
  Constant18/1 -> Relational Operator15/2
  pDCCI_st_DCDCActSt/1 -> Relational Operator15/1
  Relational Operator15/1 -> pOUTP_st_HCU10DCDCSt/1  "pOUTP_st_HCU10DCDCSt"
  pBMSI_degC_BatAvgTemp/1 -> pOUTP_degC_HCU10BatPackTemp/1  "pBMSI_degC_BatAvgTemp"
  pBMSI_st_BatIslaMeasSt/1 -> pOUTP_st_HCU10IslaWarn/1  "pBMSI_st_BatIslaMeasSt"
  pMCA_Nm_MCU1TMTorqReq/1 -> Sum/1
  pMCA_Nm_MCU2TMTorqReq/1 -> Sum/2
  pMCI_Nm_MCU1MotCtrlActTrq/1 -> Product3/1
  pMCI_rpm_MCU1MotCtrlActRev/1 -> Product3/2
  Switch/1 -> pHMI_Nm_IndicateDrvTrq/1
  Relational Operator/1 -> Switch/2
  Data Type Conversion/1 -> Switch/3, Relational Operator/2
  Constant40/1 -> Data Type Conversion/1
  Sum/1 -> Switch/1, Relational Operator/1
  pBMSI_A_BatActCurr/1 -> Convert8/1
  pBMSI_pct_BatSOC/1 -> Convert13/1  "pBMSI_pct_BatSOC"
  pSHLI_st_ECOSwtSt/1 -> pOUTP_bool_HCU10ECOSwtInd/1  "pSHLI_st_ECOSwtSt"
  Convert8/1 -> pOUTP_A_HCU10BatPackCurr/1  "pOUTP_A_HCU10BatPackCurr"
  Convert11/1 -> pOUTP_st_HCU10ChrgrSt/1
  pBMSI_st_BMSChrgSt/1 -> Convert11/1  "pBMSI_st_BMSChrgSt"
  Product3/1 -> Product4/1
  Constant54/1 -> Product4/2
  Product4/1 -> Switch4/2, Product1/1, Product2/1
  Switch4/1 -> pOUTP_pct_HCU10OutPwrPct/1
  Product1/1 -> Switch4/1
  Constant1/1 -> Product1/2
  Product2/1 -> Switch4/3
  Constant2/1 -> Product2/2
  Lookup Table/1 -> pOUTP_pct_HCU10BatPackSOC/1
  Convert13/1 -> Lookup Table/1
  s_NMHA_CanSlpCmd_na/1 -> pOUTP_bool_HCU10SleepIndSig/1
  pBMSI_st_BMSErr/1 -> GetBit1/1
  GetBit1/1 -> pOUTP_bool_HCU10IntlkSysFlt/1

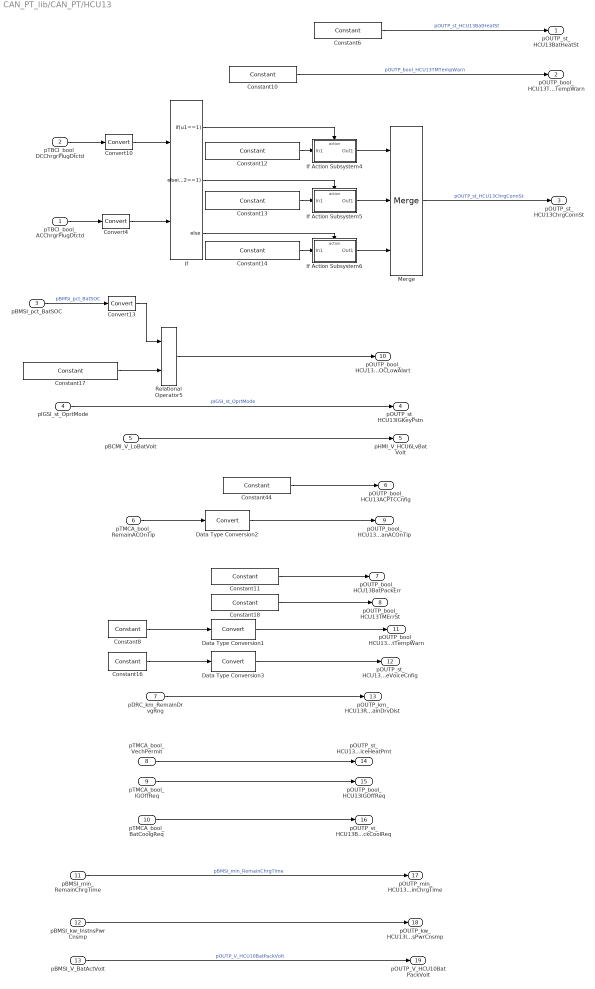
== system CAN_PT_lib/CAN_PT/HCU13 ==
  pTBCI_bool_ACChrgrPlugDtctd : Inport
  pTBCI_bool_DCChrgrPlugDtctd : Inport  Port=2
  pBMSI_pct_BatSOC : Inport  Port=3
  pIGSI_st_OprtMode : Inport  Port=4
  pBCMI_V_LoBatVolt : Inport  Port=5
  pTMCA_bool_RemainACOnTip : Inport  Port=6
  pDRC_km_RemainDrvgRng : Inport  Port=7  OutDataType=fixdt(1, 16)  OutScaling=2^0
  pTMCA_bool_VechPermit : Inport  Port=8  OutDataType=fixdt(1, 16)  OutScaling=2^0
  pTMCA_bool_IGOffReq : Inport  Port=9  OutDataType=fixdt(1, 16)  OutScaling=2^0
  pTMCA_bool_BatCoolgReq : Inport  Port=10  OutDataType=fixdt(1, 16)  OutScaling=2^0
  pBMSI_min_RemainChrgTime : Inport  Port=11
  pBMSI_kw_InstnsPwrCnsmp : Inport  Port=12
  pBMSI_V_BatActVolt : Inport  Port=13
  Constant{6,10..11,18} (4 alike) : BaseOperationLib_Browser/Sources&Sinks/Constant  Value=p_bool_False_M  OutMin=[]  OutMax=[]  OutDataType=fixdt(1, 16)  ConRadixGroup=Use specified scaling  OutScaling=2^0  OutDataTypeStr=Inherit: Inherit from 'Constant value'
  Constant12 : BaseOperationLib_Browser/Sources&Sinks/Constant  Value=pOUTP_st_ChrgrPlugStOne_C  OutMin=[]  OutMax=[]  OutDataType=fixdt(1, 16)  ConRadixGroup=Use specified scaling  OutScaling=2^0  OutDataTypeStr=Inherit: Inherit from 'Constant value'
  Constant13 : BaseOperationLib_Browser/Sources&Sinks/Constant  Value=pOUTP_st_ChrgrPlugStTwo_C  OutMin=[]  OutMax=[]  OutDataType=fixdt(1, 16)  ConRadixGroup=Use specified scaling  OutScaling=2^0  OutDataTypeStr=Inherit: Inherit from 'Constant value'
  Constant14 : BaseOperationLib_Browser/Sources&Sinks/Constant  Value=pOUTP_st_ChrgrPlugStZero_C  OutMin=[]  OutMax=[]  OutDataType=fixdt(1, 16)  ConRadixGroup=Use specified scaling  OutScaling=2^0  OutDataTypeStr=Inherit: Inherit from 'Constant value'
  Constant16 : BaseOperationLib_Browser/Sources&Sinks/Constant  Value=0  OutMin=[]  OutMax=[]  OutDataType=fixdt(1, 16)  ConRadixGroup=Use specified scaling  OutScaling=2^0  OutDataTypeStr=Inherit: Inherit from 'Constant value'
  Constant17 : BaseOperationLib_Browser/Sources&Sinks/Constant  Value=pOUTP_pct_BatSOCLim_C  OutMin=[]  OutMax=[]  OutDataType=fixdt(1, 16)  ConRadixGroup=Use specified scaling  OutScaling=2^0  OutDataTypeStr=Inherit: Inherit from 'Constant value'
  Constant44 : BaseOperationLib_Browser/Sources&Sinks/Constant  Value=pOUTP_st_ACPTCfg_C  OutMin=[]  OutMax=[]  OutDataType=fixdt(1, 16)  ConRadixGroup=Use specified scaling  OutScaling=2^0  OutDataTypeStr=Inherit: Inherit from 'Constant value'
  Constant8 : BaseOperationLib_Browser/Sources&Sinks/Constant  Value=0  OutMin=[]  OutMax=[]  OutDataType=fixdt(1, 16)  ConRadixGroup=Use specified scaling  OutScaling=2^0  OutDataTypeStr=Inherit: Inherit from 'Constant value'
  Convert10 : DataTypeConversion  OutDataType=fixdt(1, 16)  OutScaling=2^0
  Convert13 : DataTypeConversion  OutDataType=fixdt(1, 16)  OutScaling=2^0
  Convert4 : DataTypeConversion  OutDataType=fixdt(1, 16)  OutScaling=2^0
  Data Type Conversion1 : DataTypeConversion  OutDataType=fixdt(1, 16)  OutScaling=2^0
  Data Type Conversion2 : DataTypeConversion  OutDataType=fixdt(1, 16)  OutScaling=2^0
  Data Type Conversion3 : DataTypeConversion  OutDataType=fixdt(1, 16)  OutScaling=2^0
  If : If  NumInputs=2  IfExpression=u1==1  ElseIfExpressions=u2==1
  If Action Subsystem4 : Subsystem  TreatAsAtomicUnit=on
  If Action Subsystem5 : Subsystem  TreatAsAtomicUnit=on
  If Action Subsystem6 : Subsystem  TreatAsAtomicUnit=on
  Merge : Merge  Inputs=3
  Relational Operator5 : BaseOperationLib_Browser/Logic Operations Changed/Relational Operator  Operator=<  InputSameDT=on  LogicOutDataTypeMode=Specify via dialog  LogicDataType=PDT_Bool  OutDataTypeStr=PDT_Bool
  pOUTP_st_HCU13BatHeatSt : Outport
  pOUTP_bool_HCU13TMTempWarn : Outport  Port=2
  pOUTP_st_HCU13ChrgConnSt : Outport  Port=3
  pOUTP_st_HCU13IGKeyPstn : Outport  Port=4
  pHMI_V_HCU6LvBatVolt : Outport  Port=5
  pOUTP_bool_HCU13ACPTCCnfig : Outport  Port=6
  pOUTP_bool_HCU13BatPackErr : Outport  Port=7
  pOUTP_bool_HCU13TMErrSt : Outport  Port=8
  pOUTP_bool_HCU13RemanACOnTip : Outport  Port=9  OutDataType=fixdt(1, 16)  OutScaling=2^0
  pOUTP_bool_HCU13BatSOCLowAlart : Outport  Port=10
  pOUTP_bool_HCU13BatTempWarn : Outport  Port=11  OutDataType=fixdt(1, 16)  OutScaling=2^0
  pOUTP_st_HCU13NoiseVoiceCnfig : Outport  Port=12  OutDataType=fixdt(1, 16)  OutScaling=2^0
  pOUTP_km_HCU13RemainDrvDist : Outport  Port=13  OutDataType=fixdt(1, 16)  OutScaling=2^0
  pOUTP_st_HCU13VehDeiceHeatPmt : Outport  Port=14  OutDataType=fixdt(1, 16)  OutScaling=2^0
  pOUTP_bool_HCU13IGOffReq : Outport  Port=15  OutDataType=fixdt(1, 16)  OutScaling=2^0
  pOUTP_st_HCU13BatPackCoolReq : Outport  Port=16  OutDataType=fixdt(1, 16)  OutScaling=2^0
  pOUTP_min_HCU13RemainChrgTime : Outport  Port=17
  pOUTP_kw_HCU13InstnsPwrCnsmp : Outport  Port=18
  pOUTP_V_HCU10BatPackVolt : Outport  Port=19
  wires:
  pBMSI_kw_InstnsPwrCnsmp/1 -> pOUTP_kw_HCU13InstnsPwrCnsmp/1
  pBMSI_min_RemainChrgTime/1 -> pOUTP_min_HCU13RemainChrgTime/1  "pBMSI_min_RemainChrgTime"
  pBMSI_V_BatActVolt/1 -> pOUTP_V_HCU10BatPackVolt/1  "pOUTP_V_HCU10BatPackVolt"
  pTMCA_bool_VechPermit/1 -> pOUTP_st_HCU13VehDeiceHeatPmt/1
  pTMCA_bool_IGOffReq/1 -> pOUTP_bool_HCU13IGOffReq/1
  pTMCA_bool_BatCoolgReq/1 -> pOUTP_st_HCU13BatPackCoolReq/1
  pIGSI_st_OprtMode/1 -> pOUTP_st_HCU13IGKeyPstn/1  "pIGSI_st_OprtMode"
  Constant18/1 -> pOUTP_bool_HCU13TMErrSt/1
  Constant11/1 -> pOUTP_bool_HCU13BatPackErr/1
  If/3 -> If Action Subsystem6/Action
  Convert10/1 -> If/1
  Convert4/1 -> If/2
  If Action Subsystem6/1(Out1) -> Merge/3
  Constant14/1 -> If Action Subsystem6/1(In1)
  If Action Subsystem5/1(Out1) -> Merge/2
  If Action Subsystem4/1(Out1) -> Merge/1
  Constant13/1 -> If Action Subsystem5/1(In1)
  Constant12/1 -> If Action Subsystem4/1(In1)
  If/2 -> If Action Subsystem5/Action
  If/1 -> If Action Subsystem4/Action
  pTBCI_bool_ACChrgrPlugDtctd/1 -> Convert4/1
  pTBCI_bool_DCChrgrPlugDtctd/1 -> Convert10/1
  Merge/1 -> pOUTP_st_HCU13ChrgConnSt/1  "pOUTP_st_HCU13ChrgConnSt"
  Data Type Conversion2/1 -> pOUTP_bool_HCU13RemanACOnTip/1
  pTMCA_bool_RemainACOnTip/1 -> Data Type Conversion2/1
  Convert13/1 -> Relational Operator5/1
  Constant6/1 -> pOUTP_st_HCU13BatHeatSt/1  "pOUTP_st_HCU13BatHeatSt"
  pBCMI_V_LoBatVolt/1 -> pHMI_V_HCU6LvBatVolt/1
  Constant44/1 -> pOUTP_bool_HCU13ACPTCCnfig/1
  pBMSI_pct_BatSOC/1 -> Convert13/1  "pBMSI_pct_BatSOC"
  Constant10/1 -> pOUTP_bool_HCU13TMTempWarn/1  "pOUTP_bool_HCU13TMTempWarn"
  Constant17/1 -> Relational Operator5/2
  Relational Operator5/1 -> pOUTP_bool_HCU13BatSOCLowAlart/1
  Data Type Conversion3/1 -> pOUTP_st_HCU13NoiseVoiceCnfig/1
  Constant16/1 -> Data Type Conversion3/1
  Data Type Conversion1/1 -> pOUTP_bool_HCU13BatTempWarn/1
  Constant8/1 -> Data Type Conversion1/1
  pDRC_km_RemainDrvgRng/1 -> pOUTP_km_HCU13RemainDrvDist/1

== system CAN_PT_lib/CAN_PT/HCU14 ==
  pSHLA_st_ShftLvrPosnIC : Inport  OutDataType=fixdt(1, 16)  OutScaling=2^0
  pOUTP_st_HCU14LvlInfo : Outport  OutDataType=fixdt(1, 16)  OutScaling=2^0
  wires:
  pSHLA_st_ShftLvrPosnIC/1 -> pOUTP_st_HCU14LvlInfo/1

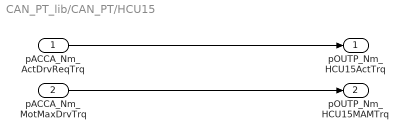
== system CAN_PT_lib/CAN_PT/HCU15 ==
  pACCA_Nm_ActDrvReqTrq : Inport  OutDataType=fixdt(1, 16)  OutScaling=2^0
  pACCA_Nm_MotMaxDrvTrq : Inport  Port=2  OutDataType=fixdt(1, 16)  OutScaling=2^0
  pOUTP_Nm_HCU15ActTrq : Outport
  pOUTP_Nm_HCU15MAMTrq : Outport  Port=2
  wires:
  pACCA_Nm_ActDrvReqTrq/1 -> pOUTP_Nm_HCU15ActTrq/1
  pACCA_Nm_MotMaxDrvTrq/1 -> pOUTP_Nm_HCU15MAMTrq/1

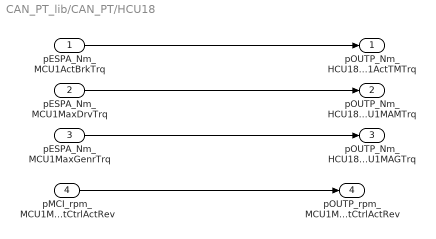
== system CAN_PT_lib/CAN_PT/HCU18 ==
  pESPA_Nm_MCU1ActBrkTrq : Inport  OutDataType=fixdt(1, 16)  OutScaling=2^0
  pESPA_Nm_MCU1MaxDrvTrq : Inport  Port=2  OutDataType=fixdt(1, 16)  OutScaling=2^0
  pESPA_Nm_MCU1MaxGenrTrq : Inport  Port=3  OutDataType=fixdt(1, 16)  OutScaling=2^0
  pMCI_rpm_MCU1MotCtrlActRev : Inport  Port=4
  pOUTP_Nm_HCU18MCU1ActTMTrq : Outport
  pOUTP_Nm_HCU18MCU1MAMTrq : Outport  Port=2
  pOUTP_Nm_HCU18MCU1MAGTrq : Outport  Port=3
  pOUTP_rpm_MCU1MotCtrlActRev : Outport  Port=4
  wires:
  pESPA_Nm_MCU1ActBrkTrq/1 -> pOUTP_Nm_HCU18MCU1ActTMTrq/1
  pESPA_Nm_MCU1MaxDrvTrq/1 -> pOUTP_Nm_HCU18MCU1MAMTrq/1
  pESPA_Nm_MCU1MaxGenrTrq/1 -> pOUTP_Nm_HCU18MCU1MAGTrq/1
  pMCI_rpm_MCU1MotCtrlActRev/1 -> pOUTP_rpm_MCU1MotCtrlActRev/1

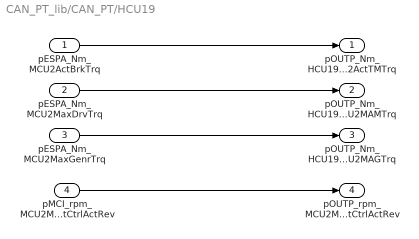
== system CAN_PT_lib/CAN_PT/HCU19 ==
  pESPA_Nm_MCU2ActBrkTrq : Inport  OutDataType=fixdt(1, 16)  OutScaling=2^0
  pESPA_Nm_MCU2MaxDrvTrq : Inport  Port=2  OutDataType=fixdt(1, 16)  OutScaling=2^0
  pESPA_Nm_MCU2MaxGenrTrq : Inport  Port=3  OutDataType=fixdt(1, 16)  OutScaling=2^0
  pMCI_rpm_MCU2MotCtrlActRev : Inport  Port=4
  pOUTP_Nm_HCU19MCU2ActTMTrq : Outport
  pOUTP_Nm_HCU19MCU2MAMTrq : Outport  Port=2
  pOUTP_Nm_HCU19MCU2MAGTrq : Outport  Port=3
  pOUTP_rpm_MCU2MotCtrlActRev : Outport  Port=4
  wires:
  pESPA_Nm_MCU2ActBrkTrq/1 -> pOUTP_Nm_HCU19MCU2ActTMTrq/1
  pESPA_Nm_MCU2MaxDrvTrq/1 -> pOUTP_Nm_HCU19MCU2MAMTrq/1
  pESPA_Nm_MCU2MaxGenrTrq/1 -> pOUTP_Nm_HCU19MCU2MAGTrq/1
  pMCI_rpm_MCU2MotCtrlActRev/1 -> pOUTP_rpm_MCU2MotCtrlActRev/1

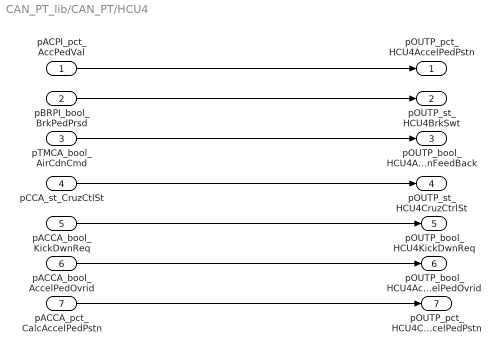
== system CAN_PT_lib/CAN_PT/HCU4 ==
  pACPI_pct_AccPedVal : Inport  OutDataType=fixdt(1, 16)  OutScaling=2^0
  pBRPI_bool_BrkPedPrsd : Inport  Port=2  OutDataType=fixdt(1, 16)  OutScaling=2^0
  pTMCA_bool_AirCdnCmd : Inport  Port=3  OutDataType=fixdt(1, 16)  OutScaling=2^0
  pCCA_st_CruzCtlSt : Inport  Port=4  OutDataType=fixdt(1, 16)  OutScaling=2^0
  pACCA_bool_KickDwnReq : Inport  Port=5  OutDataType=fixdt(1, 16)  OutScaling=2^0
  pACCA_bool_AccelPedOvrid : Inport  Port=6  OutDataType=fixdt(1, 16)  OutScaling=2^0
  pACCA_pct_CalcAccelPedPstn : Inport  Port=7  OutDataType=fixdt(1, 16)  OutScaling=2^0
  pOUTP_pct_HCU4AccelPedPstn : Outport  OutDataType=fixdt(1, 16)  OutScaling=2^0
  pOUTP_st_HCU4BrkSwt : Outport  Port=2  OutDataType=fixdt(1, 16)  OutScaling=2^0
  pOUTP_bool_HCU4ACOnFeedBack : Outport  Port=3  OutDataType=fixdt(1, 16)  OutScaling=2^0
  pOUTP_st_HCU4CruzCtrlSt : Outport  Port=4  OutDataType=fixdt(1, 16)  OutScaling=2^0
  pOUTP_bool_HCU4KickDwnReq : Outport  Port=5
  pOUTP_bool_HCU4AccelPedOvrid : Outport  Port=6
  pOUTP_pct_HCU4CalcAccelPedPstn : Outport  Port=7  OutDataType=fixdt(1, 16)  OutScaling=2^0
  wires:
  pCCA_st_CruzCtlSt/1 -> pOUTP_st_HCU4CruzCtrlSt/1
  pTMCA_bool_AirCdnCmd/1 -> pOUTP_bool_HCU4ACOnFeedBack/1
  pBRPI_bool_BrkPedPrsd/1 -> pOUTP_st_HCU4BrkSwt/1
  pACPI_pct_AccPedVal/1 -> pOUTP_pct_HCU4AccelPedPstn/1
  pACCA_bool_KickDwnReq/1 -> pOUTP_bool_HCU4KickDwnReq/1
  pACCA_bool_AccelPedOvrid/1 -> pOUTP_bool_HCU4AccelPedOvrid/1
  pACCA_pct_CalcAccelPedPstn/1 -> pOUTP_pct_HCU4CalcAccelPedPstn/1

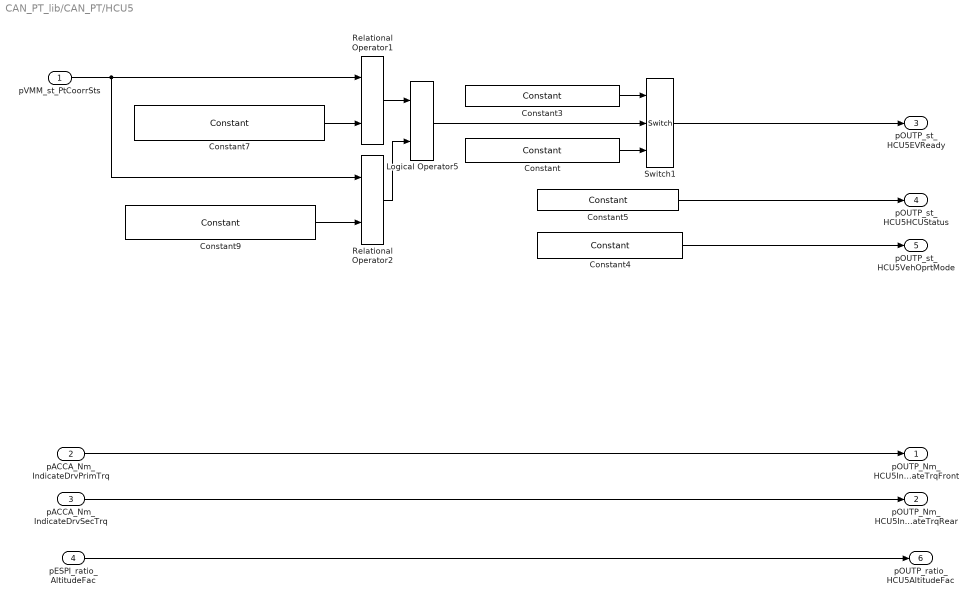
== system CAN_PT_lib/CAN_PT/HCU5 ==
  pVMM_st_PtCoorrSts : Inport
  pACCA_Nm_IndicateDrvPrimTrq : Inport  Port=2  OutDataType=fixdt(1, 16)  OutScaling=2^0
  pACCA_Nm_IndicateDrvSecTrq : Inport  Port=3  OutDataType=fixdt(1, 16)  OutScaling=2^0
  pESPI_ratio_AltitudeFac : Inport  Port=4
  Constant : BaseOperationLib_Browser/Sources&Sinks/Constant  Value=pOUTP_st_EVRdyNoSt_C  OutMin=[]  OutMax=[]  OutDataType=fixdt(1, 16)  ConRadixGroup=Use specified scaling  OutScaling=2^0  OutDataTypeStr=Inherit: Inherit from 'Constant value'
  Constant3 : BaseOperationLib_Browser/Sources&Sinks/Constant  Value=pOUTP_st_EVRdyRdySt_C  OutMin=[]  OutMax=[]  OutDataType=fixdt(1, 16)  ConRadixGroup=Use specified scaling  OutScaling=2^0  OutDataTypeStr=Inherit: Inherit from 'Constant value'
  Constant4 : BaseOperationLib_Browser/Sources&Sinks/Constant  Value=p_bool_False_M  OutMin=[]  OutMax=[]  OutDataType=fixdt(1, 16)  ConRadixGroup=Use specified scaling  OutScaling=2^0  OutDataTypeStr=Inherit: Inherit from 'Constant value'
  Constant5 : BaseOperationLib_Browser/Sources&Sinks/Constant  Value=pOUTP_st_HCUStNoErr_C  OutMin=[]  OutMax=[]  OutDataType=fixdt(1, 16)  ConRadixGroup=Use specified scaling  OutScaling=2^0  OutDataTypeStr=Inherit: Inherit from 'Constant value'
  Constant7 : BaseOperationLib_Browser/Sources&Sinks/Constant  Value=uint8(VMMCoorrStsTyp.VMM_Drv)  OutMin=[]  OutMax=[]  OutDataType=Enum: EgyCoorrStsTyp  ConRadixGroup=Best Precision: Vector-wise  OutScaling=[]  OutDataTypeStr=Inherit: Inherit from 'Constant value'
  Constant9 : BaseOperationLib_Browser/Sources&Sinks/Constant  Value=uint8(VMMCoorrStsTyp.VMM_Drv)  OutMin=[]  OutMax=[]  OutDataType=Enum: EgyCoorrStsTyp  ConRadixGroup=Best Precision: Vector-wise  OutScaling=[]  OutDataTypeStr=Inherit: Inherit from 'Constant value'
  Logical Operator5 : BaseOperationLib_Browser/Logic Operations Changed/Logical Operator  Operator=OR  Inputs=2  AllPortsSameDT=on  OutDataTypeMode=Specify via dialog  LogicDataType=PDT_Bool  OutDataTypeStr=PDT_Bool
  Relational Operator1 : BaseOperationLib_Browser/Logic Operations Changed/Relational Operator  Operator===  InputSameDT=on  LogicOutDataTypeMode=Specify via dialog  LogicDataType=PDT_Bool  OutDataTypeStr=PDT_Bool
  Relational Operator2 : BaseOperationLib_Browser/Logic Operations Changed/Relational Operator  Operator===  InputSameDT=on  LogicOutDataTypeMode=Specify via dialog  LogicDataType=PDT_Bool  OutDataTypeStr=PDT_Bool
  Switch1 : BaseOperationLib_Browser/Signal Routing Changed/Switch  Criteria=u2 ~= 0  Threshold=1  InputSameDT=on  OutMin=[]  OutMax=[]  OutDataType=fixdt(1,16,0)  OutScaling=[]  SaturateOnIntegerOverflow=on
  pOUTP_Nm_HCU5IndicateTrqFront : Outport
  pOUTP_Nm_HCU5IndicateTrqRear : Outport  Port=2
  pOUTP_st_HCU5EVReady : Outport  Port=3
  pOUTP_st_HCU5HCUStatus : Outport  Port=4
  pOUTP_st_HCU5VehOprtMode : Outport  Port=5
  pOUTP_ratio_HCU5AltitudeFac : Outport  Port=6
  wires:
  pVMM_st_PtCoorrSts/1 -> Relational Operator1/1, Relational Operator2/1
  Relational Operator2/1 -> Logical Operator5/2
  Constant9/1 -> Relational Operator2/2
  Logical Operator5/1 -> Switch1/2
  Relational Operator1/1 -> Logical Operator5/1
  Constant7/1 -> Relational Operator1/2
  Constant5/1 -> pOUTP_st_HCU5HCUStatus/1
  Constant3/1 -> Switch1/1
  Constant/1 -> Switch1/3
  Switch1/1 -> pOUTP_st_HCU5EVReady/1
  Constant4/1 -> pOUTP_st_HCU5VehOprtMode/1
  pESPI_ratio_AltitudeFac/1 -> pOUTP_ratio_HCU5AltitudeFac/1
  pACCA_Nm_IndicateDrvPrimTrq/1 -> pOUTP_Nm_HCU5IndicateTrqFront/1
  pACCA_Nm_IndicateDrvSecTrq/1 -> pOUTP_Nm_HCU5IndicateTrqRear/1

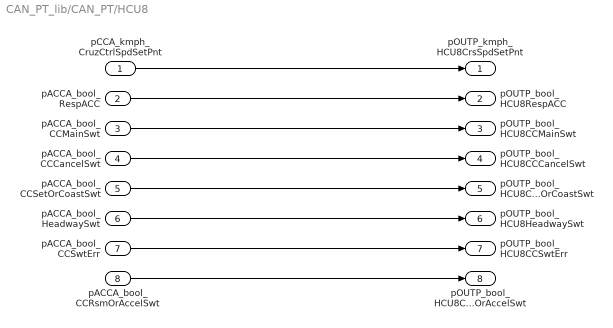
== system CAN_PT_lib/CAN_PT/HCU8 ==
  pCCA_kmph_CruzCtrlSpdSetPnt : Inport  OutDataType=fixdt(1, 16)  OutScaling=2^0
  pACCA_bool_RespACC : Inport  Port=2
  pACCA_bool_CCMainSwt : Inport  Port=3
  pACCA_bool_CCCancelSwt : Inport  Port=4
  pACCA_bool_CCSetOrCoastSwt : Inport  Port=5
  pACCA_bool_HeadwaySwt : Inport  Port=6
  pACCA_bool_CCSwtErr : Inport  Port=7
  pACCA_bool_CCRsmOrAccelSwt : Inport  Port=8
  pOUTP_kmph_HCU8CrsSpdSetPnt : Outport  OutDataType=fixdt(1, 16)  OutScaling=2^0
  pOUTP_bool_HCU8RespACC : Outport  Port=2  OutDataType=fixdt(1, 16)  OutScaling=2^0
  pOUTP_bool_HCU8CCMainSwt : Outport  Port=3  OutDataType=fixdt(1, 16)  OutScaling=2^0
  pOUTP_bool_HCU8CCCancelSwt : Outport  Port=4  OutDataType=fixdt(1, 16)  OutScaling=2^0
  pOUTP_bool_HCU8CCSetOrCoastSwt : Outport  Port=5  OutDataType=fixdt(1, 16)  OutScaling=2^0
  pOUTP_bool_HCU8HeadwaySwt : Outport  Port=6  OutDataType=fixdt(1, 16)  OutScaling=2^0
  pOUTP_bool_HCU8CCSwtErr : Outport  Port=7  OutDataType=fixdt(1, 16)  OutScaling=2^0
  pOUTP_bool_HCU8CCRsmOrAccelSwt : Outport  Port=8  OutDataType=fixdt(1, 16)  OutScaling=2^0
  wires:
  pACCA_bool_CCRsmOrAccelSwt/1 -> pOUTP_bool_HCU8CCRsmOrAccelSwt/1
  pACCA_bool_CCSwtErr/1 -> pOUTP_bool_HCU8CCSwtErr/1
  pACCA_bool_HeadwaySwt/1 -> pOUTP_bool_HCU8HeadwaySwt/1
  pACCA_bool_CCMainSwt/1 -> pOUTP_bool_HCU8CCMainSwt/1
  pACCA_bool_RespACC/1 -> pOUTP_bool_HCU8RespACC/1
  pCCA_kmph_CruzCtrlSpdSetPnt/1 -> pOUTP_kmph_HCU8CrsSpdSetPnt/1
  pACCA_bool_CCCancelSwt/1 -> pOUTP_bool_HCU8CCCancelSwt/1
  pACCA_bool_CCSetOrCoastSwt/1 -> pOUTP_bool_HCU8CCSetOrCoastSwt/1

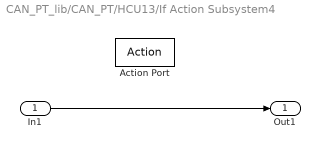
== system CAN_PT_lib/CAN_PT/HCU13/If Action Subsystem4 ==
  In1 : Inport  OutDataType=fixdt(1, 16)  OutScaling=2^0
  Action Port : ActionPort
  Out1 : Outport  OutDataType=fixdt(1, 16)  OutScaling=2^0
  wires:
  In1/1 -> Out1/1

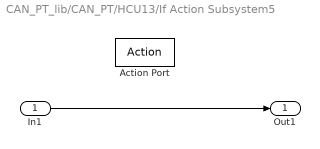
== system CAN_PT_lib/CAN_PT/HCU13/If Action Subsystem5 ==
  In1 : Inport  OutDataType=fixdt(1, 16)  OutScaling=2^0
  Action Port : ActionPort
  Out1 : Outport  OutDataType=fixdt(1, 16)  OutScaling=2^0
  wires:
  In1/1 -> Out1/1

== system CAN_PT_lib/CAN_PT/HCU13/If Action Subsystem6 ==
  In1 : Inport  OutDataType=fixdt(1, 16)  OutScaling=2^0
  Action Port : ActionPort
  Out1 : Outport  OutDataType=fixdt(1, 16)  OutScaling=2^0
  wires:
  In1/1 -> Out1/1
